simulink model "cruise_control_verification_system"  (R2024a)
settings: Solver=VariableStepAuto  StartTime=0.0  StopTime=inf  RelTol=1e-3
libraries: simulink x2
settings Model: Creator=admin  LastModifiedBy=admin

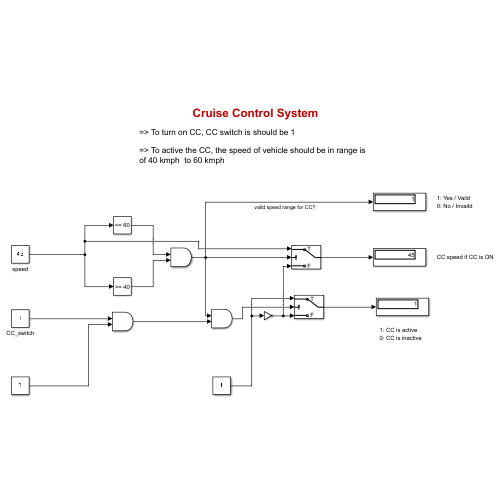
[thumbnail: Simulink's stored preview of the top-level diagram]
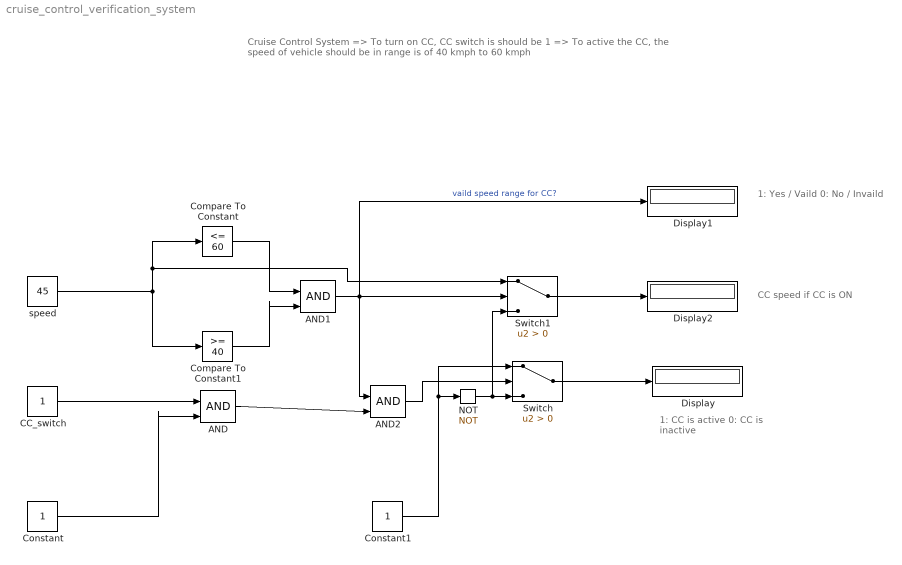
== system cruise_control_verification_system ==
  note: Cruise Control System
      |
      | => To turn on CC, CC switch is should be 1
      |
      | => To active the CC, the speed of vehicle should be in range is of 40 kmph to 60 kmph
  note: CC speed if CC is ON
  note: 1: CC is active
      | 0: CC is inactive
  note: 1: Yes / Vaild
      | 0: No / Invaild
  AND : Logic  IconShape=distinctive  AllPortsSameDT=off  OutDataTypeStr=boolean
  AND1 : Logic  IconShape=distinctive  AllPortsSameDT=off  OutDataTypeStr=boolean
  AND2 : Logic  IconShape=distinctive  AllPortsSameDT=off  OutDataTypeStr=boolean
  CC_switch : Constant
  Compare To Constant : simulink/Logic and Bit Operations/Compare To Constant  relop=<=  const=60  OutDataTypeStr=boolean
  Compare To Constant1 : simulink/Logic and Bit Operations/Compare To Constant  relop=>=  const=40  OutDataTypeStr=boolean
  Constant : Constant
  Constant1 : Constant
  Display : Display
  Display1 : Display
  Display2 : Display
  NOT : Logic  Operator=NOT  IconShape=distinctive  AllPortsSameDT=off  OutDataTypeStr=boolean
  Switch : Switch  Criteria=u2 > Threshold  SaturateOnIntegerOverflow=off  InputSameDT=off
  Switch1 : Switch  Criteria=u2 > Threshold  SaturateOnIntegerOverflow=off  InputSameDT=off
  speed : Constant  Value=45
  wires:
  Constant1/1 -> Switch/1, NOT/1
  AND1/1 -> Display1/1, Switch1/2, AND2/1  "vaild speed range for CC?"
  AND/1 -> AND2/2
  AND2/1 -> Switch/2
  Constant/1 -> AND/2
  Compare To Constant/1 -> AND1/1
  NOT/1 -> Switch1/3, Switch/3
  Switch/1 -> Display/1
  speed/1 -> Compare To Constant1/1, Compare To Constant/1, Switch1/1
  Compare To Constant1/1 -> AND1/2
  CC_switch/1 -> AND/1
  Switch1/1 -> Display2/1
